simulink model "model_v1"  (R2019b)
settings: Solver=VariableStepAuto  StartTime=0.0  StopTime=1  RelTol=1e-3
values from neighbouring files (symbols this model uses):
  phi_d = zeros(N,1)    [parameters.m]
  phi_p = zeros(N,1)    [parameters.m]
settings Model: Creator=zceeash  LastModifiedBy=zceeash

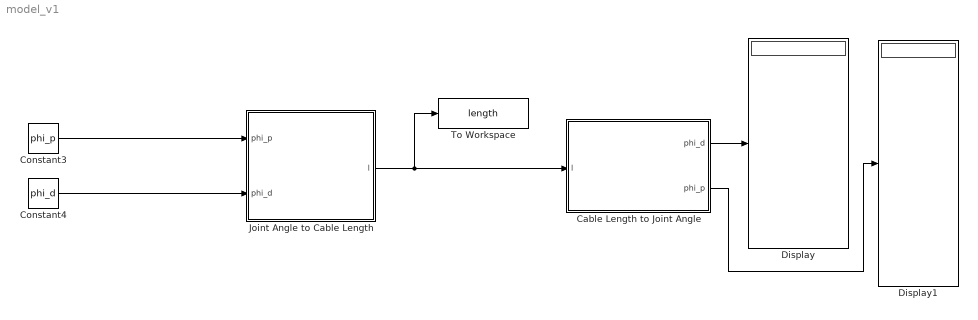
== system model_v1 ==
  " Cable Length to Joint Angle" : MATLAB Function  TreatAsAtomicUnit=on
  Constant3 : Constant  Value=phi_p
  Constant4 : Constant  Value=phi_d
  Display : Display
  Display1 : Display
  Joint Angle to Cable Length : MATLAB Function  TreatAsAtomicUnit=on
  To Workspace : ToWorkspace  VariableName=length  SampleTime=-1
  wires:
  Constant3/1 -> Joint Angle to Cable Length/1(phi_p)
  Constant4/1 -> Joint Angle to Cable Length/2(phi_d)
  " Cable Length to Joint Angle"/1(phi_d) -> Display/1
  " Cable Length to Joint Angle"/2(phi_p) -> Display1/1
  Joint Angle to Cable Length/1(l) -> " Cable Length to Joint Angle"/1(l), To Workspace/1

== matlab function model_v1/Joint Angle to Cable Length ==
  data: l output; phi_p input; phi_d input
function l = fcn(phi_p,phi_d)
N=9;
d=23/2/1000;
r=20.5/1000;
l=zeros(3*N,N);
for n=1:N
    for k=1:3*N
        if rem(n,2)==0
            delta=(12*(round((k-1)/3)+1)+120*(k-1)+90)*pi/180;
        else
            delta=(12*(round((k-1)/3)+1)+120*(k-1))*pi/180;
        end
        % delta=(360/3/n)*ceil(k/3)+360*(ceil(k/3)-1)+120*(k-3*ceil(k/3)+2);
        s_p=sin(phi_p(n));
        s_d=sin(phi_d(n));
        c_p=cos(phi_p(n));
        c_d=cos(phi_d(n));
        c_delta=cos(delta);
        s_delta=sin(delta);
        A=[ c_p        0     s_p        s_p*d;...
            s_d*s_p   c_d   -s_d*c_p   -d*s_d*c_p ;...
           -c_d*s_p   s_d    c_p*c_d    d*(c_p*c_d+1);...
            0         0      0          1];
        H=[r*c_delta;r*s_delta;0;1];
        trans_H=A*H;
        l_k_n=trans_H(1:3)-H(1:3);
        l(k,n)=abs(sqrt((l_k_n(1))^2+(l_k_n(2))^2+(l_k_n(3))^2));
    end
end

== matlab function model_v1/ Cable Length to Joint Angle ==
  data: l input; phi_d output; phi_p output
function [phi_d,phi_p] = fcn(l)
N=9;
d=23/2/1000;
r=20.5/1000;
error_tol=1/1000000;
phi_d=zeros(N,1);
phi_p=zeros(N,1);
for n=1:N
    if rem(n,2)==0
        delta_3n_0=(12*(round(((3*n)-1)/3)+1)+120*((3*n)-1)+90)*pi/180;
        delta_3n_1=(12*(round(((3*n-1)-1)/3)+1)+120*((3*n-1)-1)+90)*pi/180;
        delta_3n_2=(12*(round(((3*n-2)-1)/3)+1)+120*((3*n-2)-1)+90)*pi/180;
    else
        delta_3n_0=(12*(round(((3*n)-1)/3)+1)+120*((3*n)-1))*pi/180;
        delta_3n_1=(12*(round(((3*n-1)-1)/3)+1)+120*((3*n-1)-1))*pi/180;
        delta_3n_2=(12*(round(((3*n-2)-1)/3)+1)+120*((3*n-2)-1))*pi/180;
    end

    c_delta_3n_0=cos(delta_3n_0);
    s_delta_3n_0=sin(delta_3n_0);
    c_delta_3n_1=cos(delta_3n_1);
    s_delta_3n_1=sin(delta_3n_1);
    c_delta_3n_2=cos(delta_3n_2);
    s_delta_3n_2=sin(delta_3n_2);
   
   l_d=l(3*n-2:3*n,n);
   
   phi_j=[0;0];
   
   for j=0:1000
       s_d=sin(phi_j(1));
       s_p=sin(phi_j(2));
       c_p=cos(phi_j(2));
       c_d=cos(phi_j(1));
       l_j=[((d*s_p + r*c_p*c_delta_3n_0 - r*c_delta_3n_0)^2+...
                    (r*s_d*s_p*c_delta_3n_0 + r*c_d*s_delta_3n_0 - d*s_d*c_p - r*s_delta_3n_2)^2+...
                    (r*s_d*s_delta_3n_0 - r*c_delta_3n_0*c_d*s_p + d*c_d*c_p + d)^2)^(0.5);...
            ((d*s_p + r*c_p*c_delta_3n_0 - r*c_delta_3n_0)^2+...
                    (r*s_d*s_p*c_delta_3n_0 + r*c_d*s_delta_3n_0 - d*s_d*c_p - r*s_delta_3n_1)^2+...
                    (r*s_d*s_delta_3n_0 - r*c_delta_3n_0*c_d*s_p + d*c_d*c_p + d)^2)^(0.5);...
            ((d*s_p + r*c_p*c_delta_3n_0 - r*c_delta_3n_0)^2+...
                    (r*s_d*s_p*c_delta_3n_0 + r*c_d*s_delta_3n_0 - d*s_d*c_p - r*s_delta_3n_0)^2+...
                    (r*s_d*s_delta_3n_0 - r*c_delta_3n_0*c_d*s_p + d*c_d*c_p + d)^2)^(0.5)];
       delta_l=l_d-l_j;
       
       if (delta_l(1)<=error_tol) && (delta_l(2)<=error_tol) && (delta_l(3)<=error_tol)
           phi_d(n)=phi_j(1);
           phi_p(n)=phi_j(2);
           break;
       end
       
        dl_3n_0_dp=0.5*((d*s_p + r*c_p*c_delta_3n_0 - r*c_delta_3n_0)^2+...
                    (r*s_d*s_p*c_delta_3n_0 + r*c_d*s_delta_3n_0 - d*s_d*c_p - r*s_delta_3n_0)^2+...
                    (r*s_d*s_delta_3n_0 - r*c_delta_3n_0*c_d*s_p + d*c_d*c_p + d)^2)^(-0.5)*...
                    (2*(d*s_p + r*c_p*c_delta_3n_0 - r*c_delta_3n_0)*(d*c_p - r*s_p*c_delta_3n_0 - r*c_delta_3n_0)+...
                    2*(r*s_d*s_p*c_delta_3n_0 + r*c_d*s_delta_3n_0 - d*s_d*c_p - r*s_delta_3n_0)*(r*c_delta_3n_0*s_d*c_p + d*s_d*s_p)+...
                    2*(r*s_d*s_delta_3n_0 - r*c_delta_3n_0*c_d*s_p + d*c_d*c_p + d)*(- r*c_d*c_p*c_delta_3n_0 - d*c_d*s_p));
                
        dl_3n_0_dd=0.5*((d*s_p + r*c_p*c_delta_3n_0 - r*c_delta_3n_0)^2+...
                    (r*s_d*s_p*c_delta_3n_0 + r*c_d*s_delta_3n_0 - d*s_d*c_p - r*s_delta_3n_0)^2+...
                    (r*s_d*s_delta_3n_0 - r*c_delta_3n_0*c_d*s_p + d*c_d*c_p + d)^2)^(-0.5)*...
                    (2*(d*s_p + r*c_p*c_delta_3n_0 - r*c_delta_3n_0)*(0)+...
                    2*(r*s_d*s_p*c_delta_3n_0 + r*c_d*s_delta_3n_0 - d*s_d*c_p - r*s_delta_3n_0)*(-r*c_delta_3n_0*c_d*c_p - d*c_d*s_p)+...
                    2*(r*s_d*s_delta_3n_0 - r*c_delta_3n_0*c_d*s_p + d*c_d*c_p + d)*(r*c_d*s_delta_3n_0 + r*c_delta_3n_0*s_d*s_p - d*s_d*c_p));    
                     
        dl_3n_1_dp=0.5*((d*s_p + r*c_p*c_delta_3n_1 - r*c_delta_3n_1)^2+...
                    (r*s_d*s_p*c_delta_3n_1 + r*c_d*s_delta_3n_1 - d*s_d*c_p - r*s_delta_3n_1)^2+...
                    (r*s_d*s_delta_3n_1 - r*c_delta_3n_1*c_d*s_p + d*c_d*c_p + d)^2)^(-0.5)*...
                    (2*(d*s_p + r*c_p*c_delta_3n_1 - r*c_delta_3n_1)*(d*c_p - r*s_p*c_delta_3n_1 - r*c_delta_3n_1)+...
                     2*(r*s_d*s_p*c_delta_3n_1 + r*c_d*s_delta_3n_1 - d*s_d*c_p - r*s_delta_3n_1)*(r*c_delta_3n_1*s_d*c_p + d*s_d*s_p)+...
                     2*(r*s_d*s_delta_3n_1 - r*c_delta_3n_1*c_d*s_p + d*c_d*c_p + d)*(- r*c_d*c_p*c_delta_3n_1 - d*c_d*s_p));
                 
       dl_3n_1_dd=0.5*((d*s_p + r*c_p*c_delta_3n_1 - r*c_delta_3n_1)^2+...
                    (r*s_d*s_p*c_delta_3n_1 + r*c_d*s_delta_3n_1 - d*s_d*c_p - r*s_delta_3n_1)^2+...
                    (r*s_d*s_delta_3n_1 - r*c_delta_3n_1*c_d*s_p + d*c_d*c_p + d)^2)^(-0.5)*...
                    (2*(d*s_p + r*c_p*c_delta_3n_1 - r*c_delta_3n_1)*(0)+...
                    2*(r*s_d*s_p*c_delta_3n_1 + r*c_d*s_delta_3n_1 - d*s_d*c_p - r*s_delta_3n_1)*(-r*c_delta_3n_1*c_d*c_p - d*c_d*s_p)+...
                    2*(r*s_d*s_delta_3n_1 - r*c_delta_3n_1*c_d*s_p + d*c_d*c_p + d)*( r*c_d*s_delta_3n_1 + r*c_delta_3n_1*s_d*s_p - d*s_d*c_p));  
                
       dl_3n_2_dp=0.5*((d*s_p + r*c_p*c_delta_3n_2 - r*c_delta_3n_2)^2+...
                    (r*s_d*s_p*c_delta_3n_2 + r*c_d*s_delta_3n_2 - d*s_d*c_p - r*s_delta_3n_2)^2+...
                    (r*s_d*s_delta_3n_2 - r*c_delta_3n_2*c_d*s_p + d*c_d*c_p + d)^2)^(-0.5)*...
                    (2*(d*s_p + r*c_p*c_delta_3n_2 - r*c_delta_3n_2)*(d*c_p - r*s_p*c_delta_3n_2 - r*c_delta_3n_2)+...
                    2*(r*s_d*s_p*c_delta_3n_2 + r*c_d*s_delta_3n_2 - d*s_d*c_p - r*s_delta_3n_2)*(r*c_delta_3n_2*s_d*c_p + d*s_d*s_p)+...
                    2*(r*s_d*s_delta_3n_2 - r*c_delta_3n_2*c_d*s_p + d*c_d*c_p + d)*(-r*c_d*c_p*c_delta_3n_2 - d*c_d*s_p));
                
       dl_3n_2_dd=0.5*((d*s_p + r*c_p*c_delta_3n_2 - r*c_delta_3n_2)^2+...
                    (r*s_d*s_p*c_delta_3n_2 + r*c_d*s_delta_3n_2 - d*s_d*c_p - r*s_delta_3n_2)^2+...
                    (r*s_d*s_delta_3n_2 - r*c_delta_3n_2*c_d*s_p + d*c_d*c_p + d)^2)^(-0.5)*...
                    (2*(d*s_p + r*c_p*c_delta_3n_2 - r*c_delta_3n_2)*(0)+...
                    2*(r*s_d*s_p*c_delta_3n_2 + r*c_d*s_delta_3n_2 - d*s_d*c_p - r*s_delta_3n_2)*(-r*c_delta_3n_2*c_d*c_p - d*c_d*s_p)+...
                    2*(r*s_d*s_delta_3n_2 - r*c_delta_3n_2*c_d*s_p + d*c_d*c_p + d)*(r*c_d*s_delta_3n_2 + r*c_delta_3n_2*s_d*s_p - d*s_d*c_p));
                
       J=[dl_3n_2_dd dl_3n_2_dp;...
          dl_3n_1_dd dl_3n_1_dp;...
          dl_3n_0_dd dl_3n_0_dp];
       J_inv=pinv(J);
       
       delta_phi= J_inv*delta_l;
       phi_j=phi_j+delta_phi;
       
       if j==1000
           phi_d(n)=NaN;
           phi_p(n)=NaN;
       end
   end
   
end


%     t1=d*s_p + r*c_p*c_delta_3n_0 - r*c_delta_3n_0;
%     t2=r*s_d*s_p*c_delta_3n_0 + r*c_d*s_delta_3n_0 - d*s_d*c_p - r*s_delta_3n_0;
%     t3=r*s_d*s_delta_3n_0 - r*c_delta_3n_0*c_d*s_p + d*c_d*c_p + d;
%     t1_p=d*c_p - r*s_p*c_delta_3n_0 - r*c_delta_3n_0;
%     t2_p=r*c_delta_3n_0*s_d*c_p + d*s_d*s_p;
%     t3_p= - r*c_d*c_p*c_delta_3n_0 - d*c_d*s_p;
%     t1_d=0;
%     t2_d=-r*c_delta_3n_0*c_d*c_p - d*c_d*s_p;
%     t3_d= r*c_d*s_delta_3n_0 + r*c_delta_3n_0*s_d*s_p - d*s_d*c_p;

% dl_3n_1_dp=0.5*((t1)^2+...
%                     (t2)^2+...
%                     (t3)^2)^(-0.5)*...
%                     (2*(t1)*(t1/p)+...
%                     2*(t2)*(t2/p)+...
%                     2*(t3)*(t3/p));
%                 
% dl_3n_2_dd=0.5*((t1)^2+...
%                 (t2)^2+...
%                 (t3)^2)^(-0.5)*...
%                 (2*(t1)*(t1/d)+...
%                 2*(t2)*(t2/d)+...
%                 2*(t3)*(t3/d));

%     dl_3n_0_dp=0.5*((t1)^2+(t2)^2+(t3)^2)^(-0.5)*(2*(t1)*(t1/p)+2*(t2)*(t2/p)+2*(t3)*(t3/p));
%     dl_3n_0_dd=0.5*((t1)^2+(t2)^2+(t3)^2)^(-0.5)*(2*(t1)*(t1/d)+2*(t2)*(t2/d)+2*(t3)*(t3/d));
